simulink model "vhf_hil_model"  (R2024a)
settings: Solver=FixedStepAuto  StartTime=0.0  StopTime=9  RelTol=1e-3
PreLoadFcn:
  | run('control_bus.m')
  | addpath('.\observers','.\control')
model workspace (MAT data in the model file):
  C = 39.8
  D = 0.05
  Lc = [1.1848250893; -624.760865246]
  M = 740
  Nd = 40
  Tmax = 1000
  a = 0.015
  esc_ic = 0.1
  g = 9.807
  h = 0.577
  l = 1.917
  lf = 1.036
  lr = 0.881
  mdlWSDbList = "E:\Henrique\Poli\Mestrado\Carsim_VHF\Extensions\Simulink\tc_vhf\Dat\msgCatalogueTCS.dbc"
  omega = 100
  phi = -1.0471975512
  re = 0.284
  x0 = 200
  x_c = 90
  x_l = 10
libraries: msgCatalogueTCSlib x11, speedgoatlib_CANLIN_OfA2 x2, speedgoatlib_IO611 x1, Solver_SF x1
CloseFcn:
  | clear control_info_bus
settings Model: DataDictionary=kf_dict.sldd  Creator=henri  LastModifiedBy=Henrique Mesquita
settings SolverCC: ConcurrentTasks=on  PositivePriorityOrder=on  AutoInsertRateTranBlk=on
settings OptimizationCC: BlockReduction=off  OptimizeBlockIOStorage=off  ReuseModelBlockBuffer=off
settings DebuggingCC: TasksWithSamePriorityMsg=none  UnconnectedInputMsg=warning  UnconnectedOutputMsg=warning  UnconnectedLineMsg=warning
settings HardwareCC: ProdBitPerLong=64  ProdLongLongMode=on  ProdHWDeviceType=Intel->x86-64 (Linux 64)
settings ModelReferenceCC: EnableRefExpFcnMdlSchedulingChecks=on
settings SFSimCC: SimUserIncludeDirs="\".\\observers\""
settings RTWCC: Description=Speedgoat Real-Time Target Machine  SystemTargetFile=speedgoat.tlc  TemplateMakefile=slrealtime_default_tmf  Toolchain=Simulink Real-Time Toolchain  BuildConfiguration=Faster Runs  CodeExecutionProfiling=on  TargetLang=C++  GPUComputeCapability=3.5  DLArmComputeVersion=19.05
settings SimulinkRealTimeTargetCC: InstructionSetFMA=off  LogToMDFFile=off

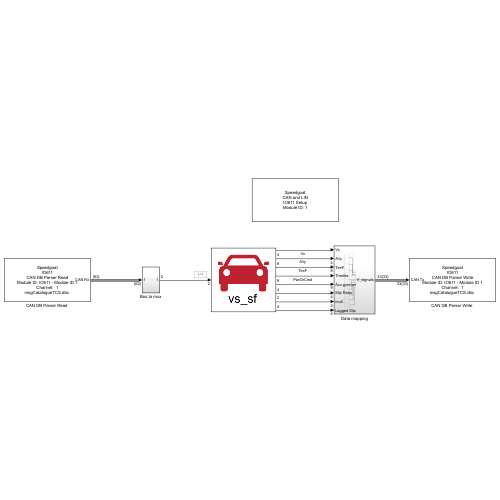
[thumbnail: Simulink's stored preview of the top-level diagram]
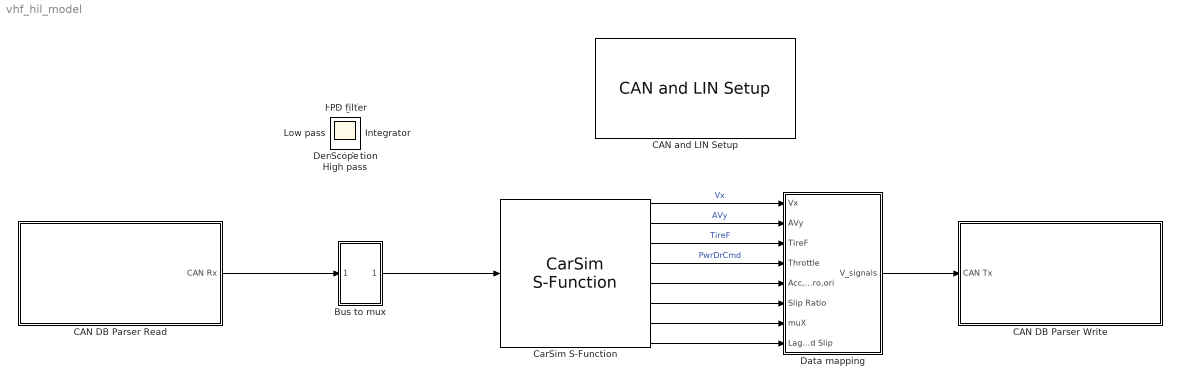
== system vhf_hil_model ==
  Bus to mux : Subsystem
  "CAN DB Parser Read " : Subsystem
      settings: OpenFcn=sg_can.OpenFcnRead;
      mask Help: eval('sg.utils.help.show(''io_main/refentry_ref_can_ofa_parsing_read'');')
      mask Display: disp('Speedgoat\nIO611\nCAN DB Parser Read\nModule ID: IO611 - Module ID 1\nChannel:  1\nmsgCatalogueTCS.dbc ');
  "CAN DB Parser Write " : Subsystem
      settings: OpenFcn=sg_can.OpenFcnWrite;
      mask Help: eval('sg.utils.help.show(''io_main/refentry_ref_can_ofa_parsing_write'');')
      mask Display: disp('Speedgoat\nIO611\nCAN DB Parser Write\nModule ID: IO611 - Module ID 1\nChannel:  1\nmsgCatalogueTCS.dbc ');
  "CAN and LIN Setup " : speedgoatlib_IO611/CAN and LIN Setup   moduleInitValues="[611    1    1   -1   -1]"  id=1  moduleType=IO611  pciSlot=-1  canChn1=CAN (HS)  canChn2=Disabled  canChn3=Disabled  canChn4=Disabled  linChn1=Disabled  linChn2=Disabled  canInitStructArray=[]  canTermStructArray=[]  canChn1InitValues="[2   4   1  31   8   2   1   5   2]"  arbBdrChn1=500 kBaud  arbManBdrChn1=[4,1,31,8]  fdBdrChn1=5.0 MBaud  fdManBdrChn1=[2,1,5,2]  canChn2InitValues="[1   2   1  31   8   2   1   5   2]"  arbBdrChn2=1.0 MBaud  arbManBdrChn2=[2,1,31,8]  fdBdrChn2=5.0 MBaud  fdManBdrChn2=[2,1,5,2]  canChn3InitValues="[1   2   1  31   8   2   1   5   2]"  arbBdrChn3=1.0 MBaud  arbManBdrChn3=[2,1,31,8]  fdBdrChn3=5.0 MBaud  fdManBdrChn3=[2,1,5,2]  canChn4InitValues="[1   2   1  31   8   2   1   5   2]"  arbBdrChn4=1.0 MBaud  arbManBdrChn4=[2,1,31,8]  fdBdrChn4=5.0 MBaud  fdManBdrChn4=[2,1,5,2]  bdrLIN1=19200  linChn1InitValues="[1  19200]"  bdrLIN2=19200  linChn2InitValues="[1  19200]"
      settings: LibrarySourceBlock=speedgoatlib_CANLIN_OfA2/CAN and LIN Setup
  CarSim S-Function : Solver_SF/CarSim S-Function  Priority=1  SIMFILE=simfile.sim  Run_RTs=off  vs_state_ind=Run  StopMode_ind=Vehicle Model
  Data mapping : Subsystem
  Demodulation : Scope
  HPF gain : Scope
  High pass : Scope
  Integrator : Scope
  Low pass : Scope
  PD filter : Scope
  Scope : Scope
  wires:
  CarSim S-Function/2 -> Data mapping/2(AVy)  "AVy"
  CarSim S-Function/6 -> Data mapping/6(Slip Ratio)
  CarSim S-Function/7 -> Data mapping/7(muX)
  CarSim S-Function/1 -> Data mapping/1(Vx)  "Vx"
  CarSim S-Function/3 -> Data mapping/3(TireF)  "TireF"
  CarSim S-Function/4 -> Data mapping/4(Throttle)  "PwrDrCmd"
  CarSim S-Function/5 -> Data mapping/5(Acc,gyro,ori)
  CarSim S-Function/8 -> Data mapping/8(Lagged Slip)
  Data mapping/1(V_signals) -> "CAN DB Parser Write "/1(CAN Tx)
  "CAN DB Parser Read "/1(CAN Rx) -> Bus to mux/1(In1)
  Bus to mux/1(Out1) -> CarSim S-Function/1

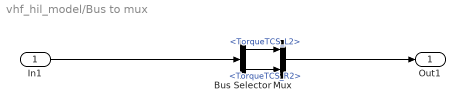
== system vhf_hil_model/Bus to mux ==
  In1 : Inport
  Bus Selector : BusSelector  OutputSignals=ID217_TorqueTCS.TorqueTCS_L2,ID217_TorqueTCS.TorqueTCS_R2
  Mux : Mux  Inputs=2
  Out1 : Outport
  wires:
  Bus Selector/2 -> Mux/2  "<TorqueTCS_R2>"
  Mux/1 -> Out1/1
  In1/1 -> Bus Selector/1
  Bus Selector/1 -> Mux/1  "<TorqueTCS_L2>"

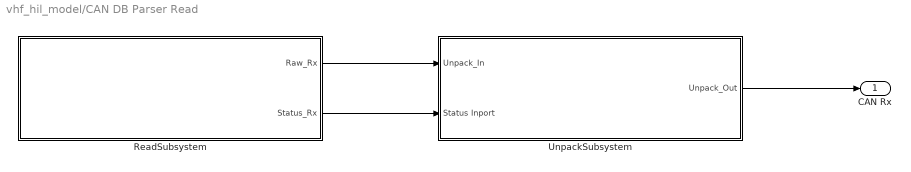
== system vhf_hil_model/CAN DB Parser Read  ==
  ReadSubsystem : Subsystem
  UnpackSubsystem : Subsystem
  CAN Rx : Outport
  wires:
  ReadSubsystem/1(Raw_Rx) -> UnpackSubsystem/1(Unpack_In)
  ReadSubsystem/2(Status_Rx) -> UnpackSubsystem/2(Status Inport)
  UnpackSubsystem/1(Unpack_Out) -> CAN Rx/1

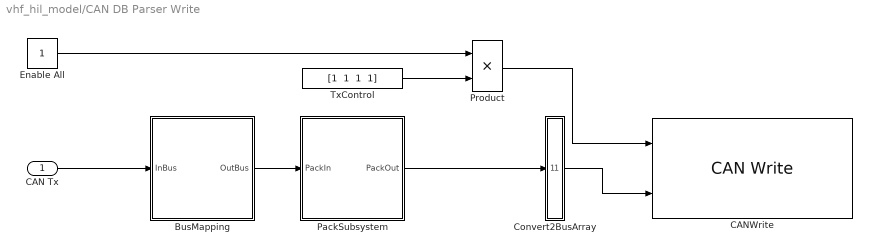
== system vhf_hil_model/CAN DB Parser Write  ==
  CAN Tx : Inport
  BusMapping : Subsystem
  CANWrite : speedgoatlib_CANLIN_OfA2/CAN/CAN Write   moduleType=IO611  id=1  channel=1  canType=CAN (HS)  useBusIn=on  numOfMsg=4  enableInput=on  enableStatusPort=off  initValues=[611 1 0.001 0 1 1 0 4 1 1]  ts=0.001
  Convert2BusArray : Subsystem
  Enable All : Constant  OutDataTypeStr=boolean
  PackSubsystem : Subsystem
  Product : Product  OutDataTypeStr=uint32
  TxControl : Constant  Value="[1  1  1  1]"  OutDataTypeStr=uint32
  wires:
  PackSubsystem/1(PackOut) -> Convert2BusArray/1(InBus)
  Convert2BusArray/1(BusArrayOut) -> CANWrite/2
  Product/1 -> CANWrite/1
  TxControl/1 -> Product/2
  Enable All/1 -> Product/1
  CAN Tx/1 -> BusMapping/1(InBus)
  BusMapping/1(OutBus) -> PackSubsystem/1(PackIn)

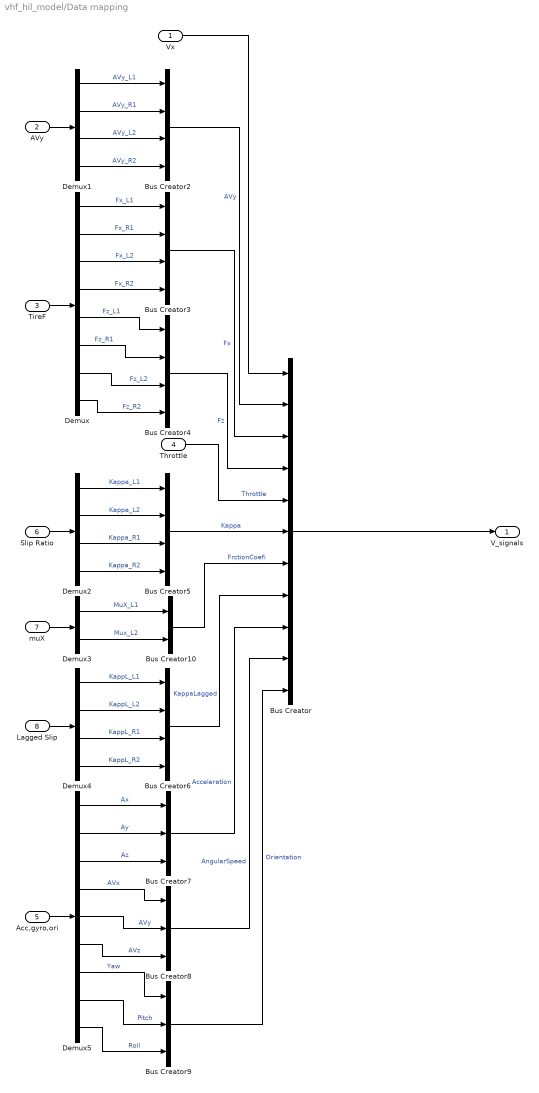
== system vhf_hil_model/Data mapping ==
  Vx : Inport
  AVy : Inport  Port=2
  TireF : Inport  Port=3
  Throttle : Inport  Port=4
  Acc,gyro,ori : Inport  Port=5
  Slip Ratio : Inport  Port=6
  muX : Inport  Port=7
  Lagged Slip : Inport  Port=8
  Bus Creator : BusCreator  Inputs=11
  Bus Creator10 : BusCreator  Inputs=2
  Bus Creator{2..6} (5 alike) : BusCreator  Inputs=4
  Bus Creator7 : BusCreator  Inputs=3
  Bus Creator8 : BusCreator  Inputs=3
  Bus Creator9 : BusCreator  Inputs=3
  Demux : Demux  Outputs=8
  Demux1 : Demux
  Demux2 : Demux
  Demux3 : Demux  Outputs=2
  Demux4 : Demux
  Demux5 : Demux  Outputs=9
  V_signals : Outport
  wires:
  Demux/8 -> Bus Creator4/4  "Fz_R2"
  Demux/6 -> Bus Creator4/2  "Fz_R1"
  Demux1/2 -> Bus Creator2/2  "AVy_R1"
  Demux/7 -> Bus Creator4/3  "Fz_L2"
  Demux/5 -> Bus Creator4/1  "Fz_L1"
  Demux1/1 -> Bus Creator2/1  "AVy_L1"
  Vx/1 -> Bus Creator/1
  AVy/1 -> Demux1/1
  Throttle/1 -> Bus Creator/5  "Throttle"
  TireF/1 -> Demux/1
  Slip Ratio/1 -> Demux2/1
  Acc,gyro,ori/1 -> Demux5/1
  Demux5/8 -> Bus Creator9/2  "Pitch"
  muX/1 -> Demux3/1
  Lagged Slip/1 -> Demux4/1
  Demux2/3 -> Bus Creator5/3  "Kappa_R1"
  Demux2/1 -> Bus Creator5/1  "Kappa_L1"
  Demux1/3 -> Bus Creator2/3  "AVy_L2"
  Demux2/4 -> Bus Creator5/4  "Kappa_R2"
  Demux2/2 -> Bus Creator5/2  "Kappa_L2"
  Demux1/4 -> Bus Creator2/4  "AVy_R2"
  Demux/3 -> Bus Creator3/3  "Fx_L2"
  Demux/1 -> Bus Creator3/1  "Fx_L1"
  Bus Creator/1 -> V_signals/1
  Demux/4 -> Bus Creator3/4  "Fx_R2"
  Demux/2 -> Bus Creator3/2  "Fx_R1"
  Demux5/3 -> Bus Creator7/3  "Az"
  Demux4/1 -> Bus Creator6/1  "KappL_L1"
  Demux3/1 -> Bus Creator10/1  "MuX_L1"
  Bus Creator5/1 -> Bus Creator/6  "Kappa"
  Demux5/4 -> Bus Creator8/1  "AVx"
  Demux4/2 -> Bus Creator6/2  "KappL_L2"
  Demux3/2 -> Bus Creator10/2  "Mux_L2"
  Demux5/1 -> Bus Creator7/1  "Ax"
  Demux4/3 -> Bus Creator6/3  "KappL_R1"
  Demux5/2 -> Bus Creator7/2  "Ay"
  Demux4/4 -> Bus Creator6/4  "KappL_R2"
  Demux5/9 -> Bus Creator9/3  "Roll"
  Demux5/5 -> Bus Creator8/2  "AVy"
  Demux5/6 -> Bus Creator8/3  "AVz"
  Demux5/7 -> Bus Creator9/1  "Yaw"
  Bus Creator2/1 -> Bus Creator/2  "AVy"
  Bus Creator3/1 -> Bus Creator/3  "Fx"
  Bus Creator4/1 -> Bus Creator/4  "Fz"
  Bus Creator10/1 -> Bus Creator/7  "FrctionCoefi"
  Bus Creator6/1 -> Bus Creator/8  "KappaLagged"
  Bus Creator7/1 -> Bus Creator/9  "Acceleration"
  Bus Creator8/1 -> Bus Creator/10  "AngularSpeed"
  Bus Creator9/1 -> Bus Creator/11  "Orientation"

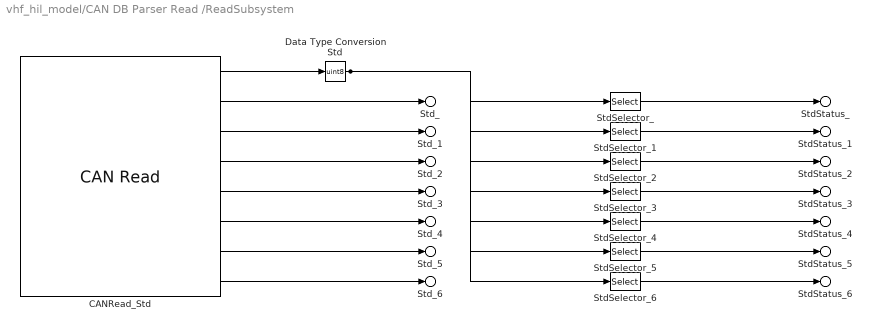
== system vhf_hil_model/CAN DB Parser Read /ReadSubsystem ==
  CANRead_Std : speedgoatlib_CANLIN_OfA2/CAN/CAN Read   moduleType=IO611  id=1  channel=1  canType=CAN (HS)  useBusOut=on  HasMulRead=Specify by IDs  MsgIDlist="[217  218  219  220  221  222  223]"  isEFF=off  LabelInHex=off  enableInput=off  ts=0.001  initValues=[611 1 0.001 0 1 1 0 1 0 2 7 217 218 219 220 221 222 223]
  Data Type ConversionStd : DataTypeConversion  OutDataTypeStr=uint8  SaturateOnIntegerOverflow=off  RndMeth=Floor
  StdSelector_ : Selector  IndexOptions=Index vector (dialog)  Indices=1  OutputSizes=1
  StdSelector_1 : Selector  IndexOptions=Index vector (dialog)  Indices=2  OutputSizes=1
  StdSelector_2 : Selector  IndexOptions=Index vector (dialog)  Indices=3  OutputSizes=1
  StdSelector_3 : Selector  IndexOptions=Index vector (dialog)  Indices=4  OutputSizes=1
  StdSelector_4 : Selector  IndexOptions=Index vector (dialog)  Indices=5  OutputSizes=1
  StdSelector_5 : Selector  IndexOptions=Index vector (dialog)  Indices=6  OutputSizes=1
  StdSelector_6 : Selector  IndexOptions=Index vector (dialog)  Indices=7  OutputSizes=1
  Std_ : Outport  PortName=Raw_Rx  Element=Std.ID217
  Std_1 : Outport  PortName=Raw_Rx  Element=Std.ID218
  Std_2 : Outport  PortName=Raw_Rx  Element=Std.ID219
  Std_3 : Outport  PortName=Raw_Rx  Element=Std.ID220
  Std_4 : Outport  PortName=Raw_Rx  Element=Std.ID221
  Std_5 : Outport  PortName=Raw_Rx  Element=Std.ID222
  Std_6 : Outport  PortName=Raw_Rx  Element=Std.ID223
  StdStatus_ : Outport  Port=2  PortName=Status_Rx  Element=Std.ID217
  StdStatus_1 : Outport  Port=2  PortName=Status_Rx  Element=Std.ID218
  StdStatus_2 : Outport  Port=2  PortName=Status_Rx  Element=Std.ID219
  StdStatus_3 : Outport  Port=2  PortName=Status_Rx  Element=Std.ID220
  StdStatus_4 : Outport  Port=2  PortName=Status_Rx  Element=Std.ID221
  StdStatus_5 : Outport  Port=2  PortName=Status_Rx  Element=Std.ID222
  StdStatus_6 : Outport  Port=2  PortName=Status_Rx  Element=Std.ID223
  wires:
  CANRead_Std/1 -> Data Type ConversionStd/1
  CANRead_Std/2 -> Std_/1
  CANRead_Std/3 -> Std_1/1
  CANRead_Std/4 -> Std_2/1
  CANRead_Std/5 -> Std_3/1
  CANRead_Std/6 -> Std_4/1
  CANRead_Std/7 -> Std_5/1
  CANRead_Std/8 -> Std_6/1
  Data Type ConversionStd/1 -> StdSelector_/1, StdSelector_1/1, StdSelector_2/1, StdSelector_3/1, StdSelector_4/1, StdSelector_5/1, StdSelector_6/1
  StdSelector_/1 -> StdStatus_/1
  StdSelector_1/1 -> StdStatus_1/1
  StdSelector_2/1 -> StdStatus_2/1
  StdSelector_3/1 -> StdStatus_3/1
  StdSelector_4/1 -> StdStatus_4/1
  StdSelector_5/1 -> StdStatus_5/1
  StdSelector_6/1 -> StdStatus_6/1

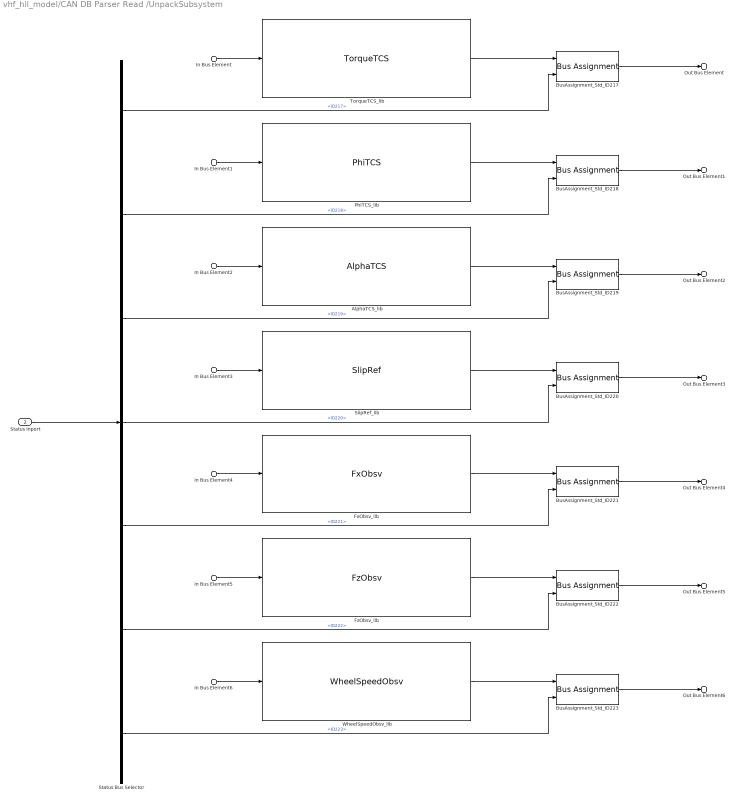
== system vhf_hil_model/CAN DB Parser Read /UnpackSubsystem ==
  In Bus Element : Inport  PortName=Unpack_In  Element=Std.ID217
  In Bus Element1 : Inport  PortName=Unpack_In  Element=Std.ID218
  In Bus Element2 : Inport  PortName=Unpack_In  Element=Std.ID219
  In Bus Element3 : Inport  PortName=Unpack_In  Element=Std.ID220
  In Bus Element4 : Inport  PortName=Unpack_In  Element=Std.ID221
  In Bus Element5 : Inport  PortName=Unpack_In  Element=Std.ID222
  In Bus Element6 : Inport  PortName=Unpack_In  Element=Std.ID223
  Status Inport : Inport  Port=2
  AlphaTCS_lib : msgCatalogueTCSlib/CAN unpack/AlphaTCS  SystemSampleTime=-1  VariantActivationTime=update diagram  AllowFlexibleInterface=on  Latency=0  AutoFrameSizeCalculation=off
  BusAssignment_Std_ID{217..223} (7 alike) : BusAssignment  AssignedSignals=MessageStatus.Status
  FxObsv_lib : msgCatalogueTCSlib/CAN unpack/FxObsv  SystemSampleTime=-1  VariantActivationTime=update diagram  AllowFlexibleInterface=on  Latency=0  AutoFrameSizeCalculation=off
  FzObsv_lib : msgCatalogueTCSlib/CAN unpack/FzObsv  SystemSampleTime=-1  VariantActivationTime=update diagram  AllowFlexibleInterface=on  Latency=0  AutoFrameSizeCalculation=off
  PhiTCS_lib : msgCatalogueTCSlib/CAN unpack/PhiTCS  SystemSampleTime=-1  VariantActivationTime=update diagram  AllowFlexibleInterface=on  Latency=0  AutoFrameSizeCalculation=off
  SlipRef_lib : msgCatalogueTCSlib/CAN unpack/SlipRef  SystemSampleTime=-1  VariantActivationTime=update diagram  AllowFlexibleInterface=on  Latency=0  AutoFrameSizeCalculation=off
  Status Bus Selector : BusSelector  OutputSignals=Std.ID217,Std.ID218,Std.ID219,Std.ID220,Std.ID221,Std.ID222,Std.ID223
  TorqueTCS_lib : msgCatalogueTCSlib/CAN unpack/TorqueTCS  SystemSampleTime=-1  VariantActivationTime=update diagram  AllowFlexibleInterface=on  Latency=0  AutoFrameSizeCalculation=off
  WheelSpeedObsv_lib : msgCatalogueTCSlib/CAN unpack/WheelSpeedObsv  SystemSampleTime=-1  VariantActivationTime=update diagram  AllowFlexibleInterface=on  Latency=0  AutoFrameSizeCalculation=off
  Out Bus Element : Outport  PortName=Unpack_Out  Element=ID217_TorqueTCS
  Out Bus Element1 : Outport  PortName=Unpack_Out  Element=ID218_PhiTCS
  Out Bus Element2 : Outport  PortName=Unpack_Out  Element=ID219_AlphaTCS
  Out Bus Element3 : Outport  PortName=Unpack_Out  Element=ID220_SlipRef
  Out Bus Element4 : Outport  PortName=Unpack_Out  Element=ID221_FxObsv
  Out Bus Element5 : Outport  PortName=Unpack_Out  Element=ID222_FzObsv
  Out Bus Element6 : Outport  PortName=Unpack_Out  Element=ID223_WheelSpeedObsv
  wires:
  In Bus Element/1 -> TorqueTCS_lib/1
  TorqueTCS_lib/1 -> BusAssignment_Std_ID217/1
  BusAssignment_Std_ID217/1 -> Out Bus Element/1
  In Bus Element1/1 -> PhiTCS_lib/1
  PhiTCS_lib/1 -> BusAssignment_Std_ID218/1
  BusAssignment_Std_ID218/1 -> Out Bus Element1/1
  In Bus Element2/1 -> AlphaTCS_lib/1
  AlphaTCS_lib/1 -> BusAssignment_Std_ID219/1
  BusAssignment_Std_ID219/1 -> Out Bus Element2/1
  In Bus Element3/1 -> SlipRef_lib/1
  SlipRef_lib/1 -> BusAssignment_Std_ID220/1
  BusAssignment_Std_ID220/1 -> Out Bus Element3/1
  In Bus Element4/1 -> FxObsv_lib/1
  FxObsv_lib/1 -> BusAssignment_Std_ID221/1
  BusAssignment_Std_ID221/1 -> Out Bus Element4/1
  In Bus Element5/1 -> FzObsv_lib/1
  FzObsv_lib/1 -> BusAssignment_Std_ID222/1
  BusAssignment_Std_ID222/1 -> Out Bus Element5/1
  In Bus Element6/1 -> WheelSpeedObsv_lib/1
  WheelSpeedObsv_lib/1 -> BusAssignment_Std_ID223/1
  BusAssignment_Std_ID223/1 -> Out Bus Element6/1
  Status Inport/1 -> Status Bus Selector/1
  Status Bus Selector/1 -> BusAssignment_Std_ID217/2  "<ID217>"
  Status Bus Selector/2 -> BusAssignment_Std_ID218/2  "<ID218>"
  Status Bus Selector/3 -> BusAssignment_Std_ID219/2  "<ID219>"
  Status Bus Selector/4 -> BusAssignment_Std_ID220/2  "<ID220>"
  Status Bus Selector/5 -> BusAssignment_Std_ID221/2  "<ID221>"
  Status Bus Selector/6 -> BusAssignment_Std_ID222/2  "<ID222>"
  Status Bus Selector/7 -> BusAssignment_Std_ID223/2  "<ID223>"

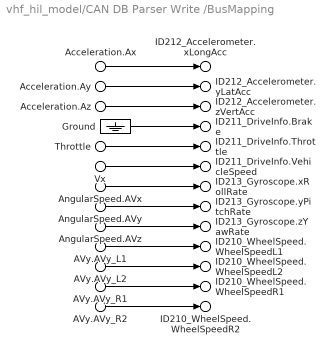
== system vhf_hil_model/CAN DB Parser Write /BusMapping ==
  Acceleration.Ax : Inport  PortName=InBus  Element=Acceleration.Ax
  Acceleration.Ay : Inport  PortName=InBus  Element=Acceleration.Ay
  Acceleration.Az : Inport  PortName=InBus  Element=Acceleration.Az
  Throttle : Inport  PortName=InBus  Element=Throttle
  Vx : Inport  PortName=InBus  Element=Vx
  AngularSpeed.AVx : Inport  PortName=InBus  Element=AngularSpeed.AVx
  AngularSpeed.AVy : Inport  PortName=InBus  Element=AngularSpeed.AVy
  AngularSpeed.AVz : Inport  PortName=InBus  Element=AngularSpeed.AVz
  AVy.AVy_L1 : Inport  PortName=InBus  Element=AVy.AVy_L1
  AVy.AVy_L2 : Inport  PortName=InBus  Element=AVy.AVy_L2
  AVy.AVy_R1 : Inport  PortName=InBus  Element=AVy.AVy_R1
  AVy.AVy_R2 : Inport  PortName=InBus  Element=AVy.AVy_R2
  Ground : Ground
  ID212_Accelerometer.xLongAcc : Outport  PortName=OutBus  Element=ID212_Accelerometer.xLongAcc
  ID212_Accelerometer.yLatAcc : Outport  PortName=OutBus  Element=ID212_Accelerometer.yLatAcc
  ID212_Accelerometer.zVertAcc : Outport  PortName=OutBus  Element=ID212_Accelerometer.zVertAcc
  ID211_DriveInfo.Brake : Outport  PortName=OutBus  Element=ID211_DriveInfo.Brake
  ID211_DriveInfo.Throttle : Outport  PortName=OutBus  Element=ID211_DriveInfo.Throttle
  ID211_DriveInfo.VehicleSpeed : Outport  PortName=OutBus  Element=ID211_DriveInfo.VehicleSpeed
  ID213_Gyroscope.xRollRate : Outport  PortName=OutBus  Element=ID213_Gyroscope.xRollRate
  ID213_Gyroscope.yPitchRate : Outport  PortName=OutBus  Element=ID213_Gyroscope.yPitchRate
  ID213_Gyroscope.zYawRate : Outport  PortName=OutBus  Element=ID213_Gyroscope.zYawRate
  ID210_WheelSpeed.WheelSpeedL1 : Outport  PortName=OutBus  Element=ID210_WheelSpeed.WheelSpeedL1
  ID210_WheelSpeed.WheelSpeedL2 : Outport  PortName=OutBus  Element=ID210_WheelSpeed.WheelSpeedL2
  ID210_WheelSpeed.WheelSpeedR1 : Outport  PortName=OutBus  Element=ID210_WheelSpeed.WheelSpeedR1
  ID210_WheelSpeed.WheelSpeedR2 : Outport  PortName=OutBus  Element=ID210_WheelSpeed.WheelSpeedR2
  wires:
  Acceleration.Ax/1 -> ID212_Accelerometer.xLongAcc/1
  Acceleration.Ay/1 -> ID212_Accelerometer.yLatAcc/1
  Acceleration.Az/1 -> ID212_Accelerometer.zVertAcc/1
  Ground/1 -> ID211_DriveInfo.Brake/1
  Throttle/1 -> ID211_DriveInfo.Throttle/1
  Vx/1 -> ID211_DriveInfo.VehicleSpeed/1
  AngularSpeed.AVx/1 -> ID213_Gyroscope.xRollRate/1
  AngularSpeed.AVy/1 -> ID213_Gyroscope.yPitchRate/1
  AngularSpeed.AVz/1 -> ID213_Gyroscope.zYawRate/1
  AVy.AVy_L1/1 -> ID210_WheelSpeed.WheelSpeedL1/1
  AVy.AVy_L2/1 -> ID210_WheelSpeed.WheelSpeedL2/1
  AVy.AVy_R1/1 -> ID210_WheelSpeed.WheelSpeedR1/1
  AVy.AVy_R2/1 -> ID210_WheelSpeed.WheelSpeedR2/1

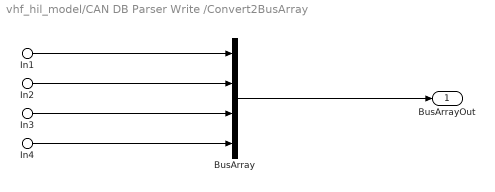
== system vhf_hil_model/CAN DB Parser Write /Convert2BusArray ==
  In1 : Inport  PortName=InBus  Element=ID210_WheelSpeed
  In2 : Inport  PortName=InBus  Element=ID211_DriveInfo
  In3 : Inport  PortName=InBus  Element=ID212_Accelerometer
  In4 : Inport  PortName=InBus  Element=ID213_Gyroscope
  BusArray : Concatenate  NumInputs=4
  BusArrayOut : Outport
  wires:
  In1/1 -> BusArray/1
  In2/1 -> BusArray/2
  In3/1 -> BusArray/3
  In4/1 -> BusArray/4
  BusArray/1 -> BusArrayOut/1

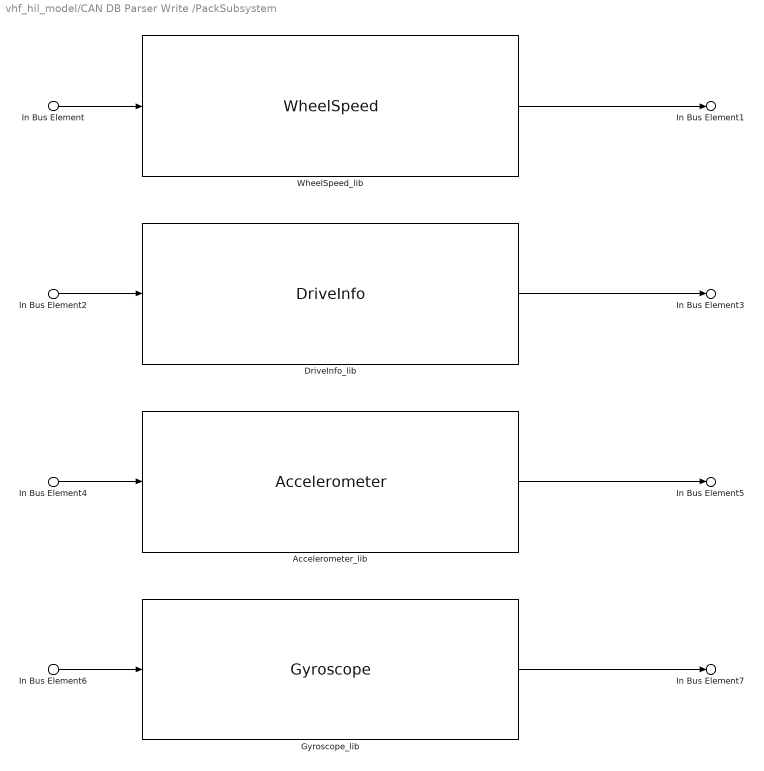
== system vhf_hil_model/CAN DB Parser Write /PackSubsystem ==
  In Bus Element : Inport  PortName=PackIn  Element=ID210_WheelSpeed
  In Bus Element2 : Inport  PortName=PackIn  Element=ID211_DriveInfo
  In Bus Element4 : Inport  PortName=PackIn  Element=ID212_Accelerometer
  In Bus Element6 : Inport  PortName=PackIn  Element=ID213_Gyroscope
  Accelerometer_lib : msgCatalogueTCSlib/CAN pack/Accelerometer  SystemSampleTime=-1  VariantActivationTime=update diagram  AllowFlexibleInterface=on  Latency=0  AutoFrameSizeCalculation=off
  DriveInfo_lib : msgCatalogueTCSlib/CAN pack/DriveInfo  SystemSampleTime=-1  VariantActivationTime=update diagram  AllowFlexibleInterface=on  Latency=0  AutoFrameSizeCalculation=off
  Gyroscope_lib : msgCatalogueTCSlib/CAN pack/Gyroscope  SystemSampleTime=-1  VariantActivationTime=update diagram  AllowFlexibleInterface=on  Latency=0  AutoFrameSizeCalculation=off
  WheelSpeed_lib : msgCatalogueTCSlib/CAN pack/WheelSpeed  SystemSampleTime=-1  VariantActivationTime=update diagram  AllowFlexibleInterface=on  Latency=0  AutoFrameSizeCalculation=off
  In Bus Element1 : Outport  PortName=PackOut  Element=ID210_WheelSpeed
  In Bus Element3 : Outport  PortName=PackOut  Element=ID211_DriveInfo
  In Bus Element5 : Outport  PortName=PackOut  Element=ID212_Accelerometer
  In Bus Element7 : Outport  PortName=PackOut  Element=ID213_Gyroscope
  wires:
  In Bus Element/1 -> WheelSpeed_lib/1
  WheelSpeed_lib/1 -> In Bus Element1/1
  In Bus Element2/1 -> DriveInfo_lib/1
  DriveInfo_lib/1 -> In Bus Element3/1
  In Bus Element4/1 -> Accelerometer_lib/1
  Accelerometer_lib/1 -> In Bus Element5/1
  In Bus Element6/1 -> Gyroscope_lib/1
  Gyroscope_lib/1 -> In Bus Element7/1
